simulink model "t6_4_Vectorizacion_2orden"  (R2024a)
settings: Solver=ode4  StartTime=0.0  StopTime=5  FixedStep=.01  RelTol=1e-3
InitFcn:
  | %wn = 10;
  | %xi = 0;
model workspace (MATLAB code in the model file):
  | % Parámetros del modelo:
  | wn = 10;
  | xi = 0;
settings Model: Creator=scpmoxxa  LastModifiedBy=scpmoxxa
settings DataIOCC: SaveFormat=Array  SaveState=on
settings OptimizationCC: ReuseModelBlockBuffer=off
settings RTWCC: GPUComputeCapability=3.5

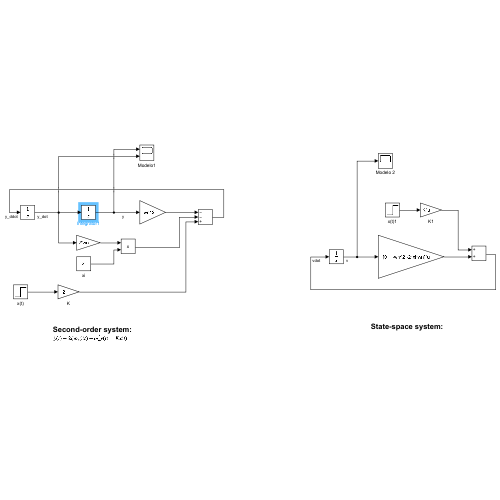
[thumbnail: Simulink's stored preview of the top-level diagram]
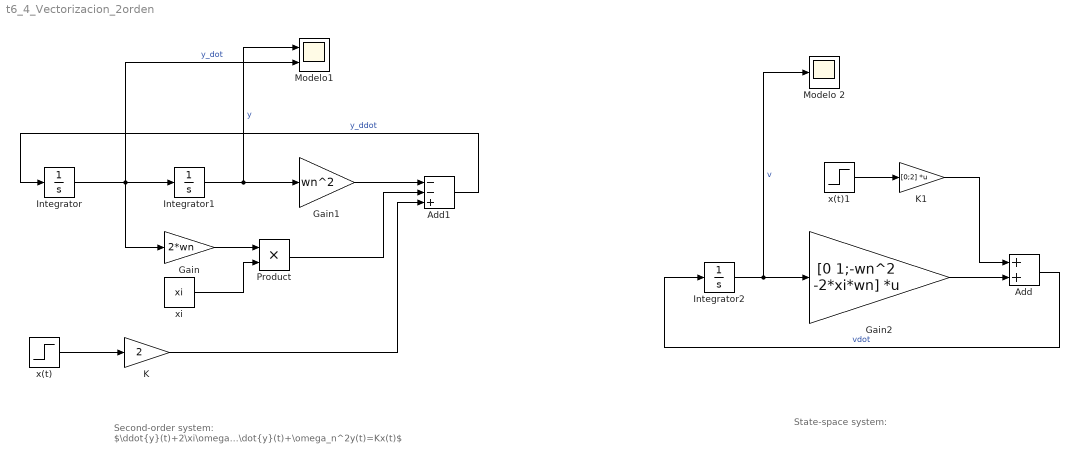
== system t6_4_Vectorizacion_2orden ==
  note: Second-order system:
      | $\ddot{y}(t)+2\xi\omega_n\dot{y}(t)+\omega_n^2y(t)=Kx(t)$
  note: State-space system:
  Add : Sum
  Add1 : Sum  Inputs=--+
  Gain : Gain  Gain=2*wn
  Gain1 : Gain  Gain=wn^2
  Gain2 : Gain  Gain=[0 1;-wn^2 -2*xi*wn]  Multiplication=Matrix(K*u)
  Integrator : Integrator
  Integrator1 : Integrator  InitialCondition=1
  Integrator2 : Integrator  InitialCondition=[1;0]
  K : Gain  Gain=2
  K1 : Gain  Gain=[0;2]  Multiplication=Matrix(K*u)
  Modelo 2 : Scope
  Modelo1 : Scope  NumInputPorts=2
  Product : Product
  x(t) : Step  SampleTime=0
  x(t)1 : Step  SampleTime=0
  xi : Constant  Value=xi
  wires:
  Add1/1 -> Integrator/1  "y_ddot"
  Integrator1/1 -> Modelo1/1, Gain1/1  "y"
  Integrator/1 -> Modelo1/2, Gain/1, Integrator1/1  "y_dot"
  Gain1/1 -> Add1/1
  K/1 -> Add1/3
  Gain/1 -> Product/1
  xi/1 -> Product/2
  Product/1 -> Add1/2
  Integrator2/1 -> Modelo 2/1, Gain2/1  "v"
  K1/1 -> Add/1
  Gain2/1 -> Add/2
  Add/1 -> Integrator2/1  "vdot"
  x(t)/1 -> K/1
  x(t)1/1 -> K1/1
